simulink model "freeSimulation"  (R2018a)
settings: Solver=FixedStepAuto  StartTime=0.0  StopTime=inf  FixedStep=1/60  RelTol=1e-3  EnableMultiTasking=on
undefined symbols (not defined in the file): Earth, WGS84
libraries: aerolibfltsims x3, aerolibanimutils x3, aerolibconvert2 x2, simulink_extras x2, aerolibtransform2 x1
settings Model: Creator=fidel  LastModifiedBy=fidel
settings DataIOCC: LimitDataPoints=on
settings OptimizationCC: LifeSpan=inf
settings DebuggingCC: AllowSymbolicDim=off  SFUnexpectedBacktrackingDiag=warning  SFNoUnconditionalDefaultTransitionDiag=warning  SFExecutionAtInitializationDiag=none
settings ModelReferenceCC: PropagateSignalLabelsOutOfModel=off
settings CodeAppCC: StateflowObjectComments=on
settings GRTTargetCC: TargetLangStandard=C89/C90 (ANSI)
settings ConfigComp: CovMetricSettings=dw  CovHtmlReporting=on  CovSaveCumulativeToWorkspaceVar=on  CovSaveSingleToWorkspaceVar=on  CovExternalEMLEnable=off

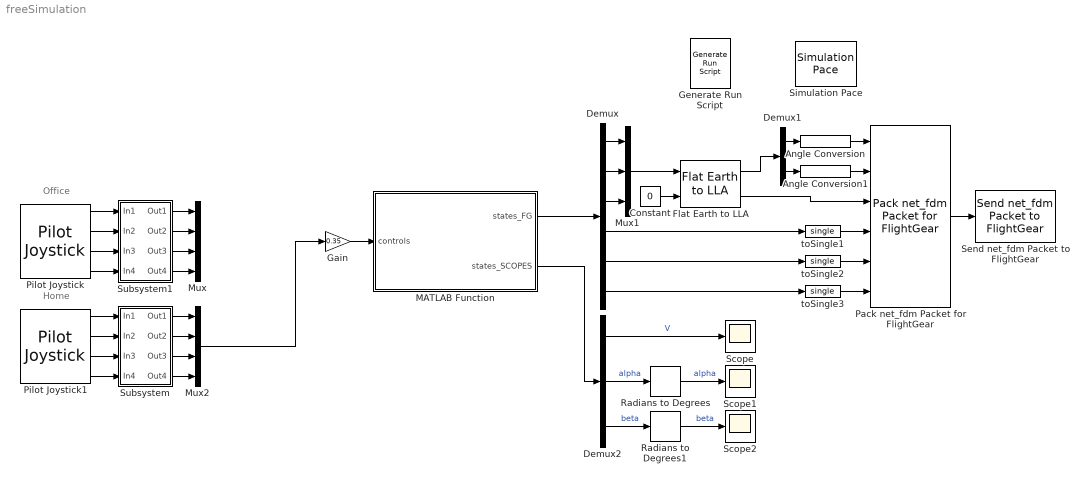
== system freeSimulation ==
  note: Office
  note: Home
  Angle Conversion : aerolibconvert2/Angle Conversion  IU=deg  OU=rad
  Angle Conversion1 : aerolibconvert2/Angle Conversion  IU=deg  OU=rad
  Constant : Constant  Value=0
  Demux : Demux  Outputs=6
  Demux1 : Demux  Outputs=2
  Demux2 : Demux  Outputs=3
  Flat Earth to LLA : aerolibtransform2/Flat Earth to LLA  units=Metric (MKS)  ptype=Earth (WGS84)  F=1/298.257223563  R=6378137  LL0=[0 10]  psi=90
  Gain : Gain  Gain=0.35
  Generate Run Script : aerolibfltsims/Generate Run Script  Architecture=Default  dataFlow=Send  GeometryModelName=ZivkoEdge540  AirportId=KSFO  RunwayId=10L  InitialAltitude=7224  InitialHeading=113  OffsetDistance=4.72  OffsetAzimuth=0  InstallScenery=off  DisableShaders=off  OriginAddress=127.0.0.1  DestinationPort=5502  OriginPort=5505  LocalAddress=127.0.0.1  OutputFileName=optimFP_runFG.bat  FlightGearBaseDirectory=C:\Program Files\FlightGear 2016.4.4
  MATLAB Function : MATLAB Function  TreatAsAtomicUnit=on
  Mux : Mux
  Mux1 : Mux  Inputs=3
  Mux2 : Mux
  Pack net_fdm Packet for FlightGear : aerolibfltsims/Pack net_fdm Packet for FlightGear  FlightGearVersion=v3.4  ShowPositionAttitudeInputs=on  ShowVelocityAccelerationInputs=off  ShowControlSurfacePositionInputs=off  ShowEngineFuelInputs=off  ShowLandingGearInputs=off  ShowEnvironmentInputs=off  SampleTime=-1
      settings: SourceProductName=Aerospace Blockset  SourceProductBaseCode=AE
  Pilot Joystick : aerolibanimutils/Pilot Joystick  JoystickID=Joystick1  OutputConfiguration=FourAxis  SampleTime=1/60
  Pilot Joystick1 : aerolibanimutils/Pilot Joystick  JoystickID=Joystick1  OutputConfiguration=FourAxis  SampleTime=1/60
  Radians to Degrees : simulink_extras/Transformations/Radians to Degrees
  Radians to Degrees1 : simulink_extras/Transformations/Radians to Degrees
  Scope : Scope
  Scope1 : Scope
  Scope2 : Scope
  Send net_fdm Packet to FlightGear : aerolibfltsims/Send net_fdm Packet to FlightGear  DestinationIpAddress=127.0.0.1  DestinationPort=5502  LocalIpPort=-1  varLen=off  SampleTime=-1
      settings: SourceProductName=Aerospace Blockset  SourceProductBaseCode=AE
  Simulation Pace : aerolibanimutils/Simulation Pace  SimulationPace=1  SleepMode=MATLAB Thread  OutputPaceError=off  SampleTime=-1
      settings: AttributesFormatString=%<SimulationPace> sec/sec
  Subsystem : Subsystem
  Subsystem1 : Subsystem
  toSingle1 : DataTypeConversion  OutDataTypeStr=single
  toSingle2 : DataTypeConversion  OutDataTypeStr=single
  toSingle3 : DataTypeConversion  OutDataTypeStr=single
  wires:
  Angle Conversion1/1 -> Pack net_fdm Packet for FlightGear/2
  Angle Conversion/1 -> Pack net_fdm Packet for FlightGear/1
  toSingle3/1 -> Pack net_fdm Packet for FlightGear/6
  toSingle2/1 -> Pack net_fdm Packet for FlightGear/5
  toSingle1/1 -> Pack net_fdm Packet for FlightGear/4
  Pack net_fdm Packet for FlightGear/1 -> Send net_fdm Packet to FlightGear/1
  Demux/6 -> toSingle3/1
  Demux/1 -> Mux1/1
  Demux/2 -> Mux1/2
  Demux/3 -> Mux1/3
  Demux/4 -> toSingle1/1
  Demux/5 -> toSingle2/1
  Mux2/1 -> Gain/1
  MATLAB Function/1(states_FG) -> Demux/1
  Flat Earth to LLA/1 -> Demux1/1
  Flat Earth to LLA/2 -> Pack net_fdm Packet for FlightGear/3
  Mux1/1 -> Flat Earth to LLA/1
  Demux1/1 -> Angle Conversion/1
  Demux1/2 -> Angle Conversion1/1
  Constant/1 -> Flat Earth to LLA/2
  Gain/1 -> MATLAB Function/1("controls ")
  MATLAB Function/2(states_SCOPES) -> Demux2/1
  Demux2/1 -> Scope/1  "V"
  Demux2/2 -> Radians to Degrees/1  "alpha"
  Demux2/3 -> Radians to Degrees1/1  "beta"
  Radians to Degrees/1 -> Scope1/1  "alpha"
  Radians to Degrees1/1 -> Scope2/1  "beta"
  Pilot Joystick1/1 -> Subsystem/1(In1)
  Pilot Joystick1/2 -> Subsystem/2(In2)
  Pilot Joystick1/3 -> Subsystem/3(In3)
  Pilot Joystick1/4 -> Subsystem/4(In4)
  Subsystem/1(Out1) -> Mux2/1
  Subsystem/2(Out2) -> Mux2/2
  Subsystem/3(Out3) -> Mux2/3
  Subsystem/4(Out4) -> Mux2/4
  Pilot Joystick/1 -> Subsystem1/1(In1)
  Pilot Joystick/2 -> Subsystem1/2(In2)
  Pilot Joystick/3 -> Subsystem1/3(In3)
  Pilot Joystick/4 -> Subsystem1/4(In4)
  Subsystem1/1(Out1) -> Mux/1
  Subsystem1/2(Out2) -> Mux/2
  Subsystem1/3(Out3) -> Mux/3
  Subsystem1/4(Out4) -> Mux/4

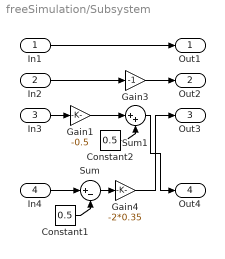
== system freeSimulation/Subsystem ==
  In1 : Inport
  In2 : Inport  Port=2
  In3 : Inport  Port=3
  In4 : Inport  Port=4
  Constant1 : Constant  Value=0.5
  Constant2 : Constant  Value=0.5
  Gain1 : Gain  Gain=-0.5
  Gain3 : Gain  Gain=-1
  Gain4 : Gain  Gain=-2*0.35
  Sum : Sum  Inputs=|+-
  Sum1 : Sum  Inputs=|++
  Out1 : Outport
  Out2 : Outport  Port=2
  Out3 : Outport  Port=3
  Out4 : Outport  Port=4
  wires:
  In4/1 -> Sum/1
  Constant1/1 -> Sum/2
  Constant2/1 -> Sum1/2
  Gain3/1 -> Out2/1
  Sum/1 -> Gain4/1
  In2/1 -> Gain3/1
  In1/1 -> Out1/1
  Gain4/1 -> Out3/1
  In3/1 -> Gain1/1
  Sum1/1 -> Out4/1
  Gain1/1 -> Sum1/1

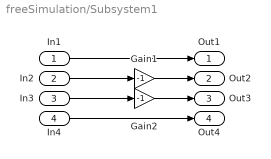
== system freeSimulation/Subsystem1 ==
  In1 : Inport
  In2 : Inport  Port=2
  In3 : Inport  Port=3
  In4 : Inport  Port=4
  Gain1 : Gain  Gain=-1
  Gain2 : Gain  Gain=-1
  Out1 : Outport
  Out2 : Outport  Port=2
  Out3 : Outport  Port=3
  Out4 : Outport  Port=4
  wires:
  In3/1 -> Gain2/1
  Gain1/1 -> Out2/1
  In4/1 -> Out4/1
  Gain2/1 -> Out3/1
  In1/1 -> Out1/1
  In2/1 -> Gain1/1

== matlab function freeSimulation/MATLAB Function ==
  data: controls input; states_FG output; states_SCOPES output
function [states_FG,states_SCOPES]  = fcn(controls)

    da = controls(1);
    de = controls(2);
    dr = controls(3);
    dt = controls(4);
    
    persistent vx;
    persistent vy;
    persistent vz;
    persistent roll;
    persistent pitch;
    persistent yaw;
    persistent p;
    persistent q;
    persistent r;
    persistent x;
    persistent y;
    persistent h;
    
    persistent dtime;
    persistent m;
    persistent g;
    persistent rho;
    persistent S;
    persistent Tmax;
    persistent b;
    persistent c;
    persistent Cd0;
    persistent Cda2;
    persistent Cdb;
    persistent Cyb;
    persistent Cyda;
    persistent Cydr;
    persistent Cyp;
    persistent Cyr;
    persistent Cl0;
    persistent Cla;
    persistent Cllb;
    persistent Cllda;
    persistent Clldr;
    persistent Cllp;
    persistent Cllr;
    persistent Cmm0;
    persistent Cmma;
    persistent Cmmda;
    persistent Cmmde;
    persistent Cmmdr;
    persistent Cmmq;
    persistent Cnnb;
    persistent Cnnda;
    persistent Cnndr;
    persistent Cnnp;
    persistent Cnnr;
    persistent Ix;
    persistent Iy;
    persistent Iz;
    persistent Ixz;
    
    if isempty(dtime)
        vx = 100;
        vy = 0;
        vz = 0;
        roll = 0;
        pitch = 0;
        yaw = 0;
        p = 0;
        q = 0;
        r = 0;
        x = 0;
        y = 0;
        h = 500;
    
        dtime = 1/60; % s
        m = 750; % kg
        g = 9.8056; % m/s^2
        rho = 1.225; % kg/m^3
        S = 9.84; % m^2
        Tmax = 16000; % N
        b = 7.87; % m
        c = S./b; % m
        Cd0 = 0.05;
        Cda2 = 0.01;
        Cdb = 0.15;
        Cyb = -0.4;
        Cyda = 0;
        Cydr = 0.19;
        Cyp = 0;
        Cyr = 0.4;
        Cl0 = 0.1205;
        Cla = 5.7;
        Cllb = -0.0002;
        Cllda = 0.33;
        Clldr = 0.021;
        Cllp = -0.79;
        Cllr = 0.075;
        Cmm0 = 0;
        Cmma = -1.23;
        Cmmda = 0;
        Cmmde = -1.1;
        Cmmdr = 0;
        Cmmq = -7.34;
        Cnnb = 0.21;
        Cnnda = -0.014;
        Cnndr = -0.11;
        Cnnp = -0.024;
        Cnnr = -0.265;
        Ix = 3531.9; % kg*m^2
        Iy = 2196.4; % kg*m^2
        Iz = 4887.7; % kg*m^2
        Ixz = 0; % kg*m^3
    end

    [V,alpha,beta] = dyn_alphaBeta(vx,vy,vz);
    [cr,sr,cp,sp,tp,cy,sy] = dyn_eulTrigon(roll,pitch,yaw);
    [coeffA,coeffB] = dyn_coeffsAux(b,c,V);
    Cd = dyn_dragCoeff(Cd0,Cda2,Cdb,alpha,beta);
    Cy = dyn_lateralForceCoeff(Cyb,Cydr,Cyda,Cyp,Cyr,beta,dr,da,coeffA,p,r);
    Cl = dyn_liftCoeff(Cl0,Cla,alpha);
    Cll = dyn_rollingMomentCoeff(Cllb,Cllda,Clldr,Cllp,Cllr,beta,da,dr,coeffA,p,r);
    Cmm = dyn_pitchingMomentCoeff(Cmm0,Cmma,Cmmde,Cmmdr,Cmmda,Cmmq,alpha,de,dr,da,coeffB,q);
    Cnn = dyn_yawingMomentCoeff(Cnnb,Cnnda,Cnndr,Cnnp,Cnnr,beta,da,dr,coeffA,p,r);
    [D,Y,L,LL,MM,NN] = dyn_forcesMomentsWind(rho,V,S,b,c,Cd,Cy,Cl,Cll,Cmm,Cnn);
    [Xa,Ya,Za,Xt] = dyn_forcesBody(alpha,beta,D,Y,L,Tmax,dt);
    [vx_dot,vy_dot,vz_dot] = dyn_velBodyDot(vx,vy,vz,p,q,r,Xa,Xt,Ya,Za,g,m,sp,cp,sr,cr);
    [roll_dot,pitch_dot,yaw_dot] = dyn_eulDot(p,q,r,tp,sr,cr,cp);
    [p_dot,q_dot,r_dot] = dyn_angularRatesDot(Ix,Iy,Iz,Ixz,p,q,r,LL,MM,NN);
    [x_dot,y_dot,h_dot] = dyn_posDot(vx,vy,vz,sr,cr,sp,cp,sy,cy);
    
    vx = vx + vx_dot*dtime;
    vy = vy + vy_dot*dtime;
    vz = vz + vz_dot*dtime;
    roll = roll + roll_dot*dtime;
    pitch = pitch + pitch_dot*dtime;
    yaw = yaw + yaw_dot*dtime;
    p = p + p_dot*dtime;
    q = q + q_dot*dtime;
    r = r + r_dot*dtime;
    x = x + x_dot*dtime;
    y = y + y_dot*dtime;
    h = h + h_dot*dtime;

    states_FG = [x;-y;-h;roll;pitch;yaw];
    states_SCOPES = [V;alpha;beta];
